simulink model "final_4_simu_20241216"  (R2021a)
settings: Solver=VariableStepAuto  StartTime=0.0  StopTime=30  RelTol=1e-3
model workspace (MAT data in the model file):
  x1_o = 0
values from neighbouring files (symbols this model uses):
  K = K_amp(1:3)    [plantilla_sscontrol.m]
  K_i = -K_amp(end)    [plantilla_sscontrol.m]
settings Model: Creator=juand  LastModifiedBy=frand

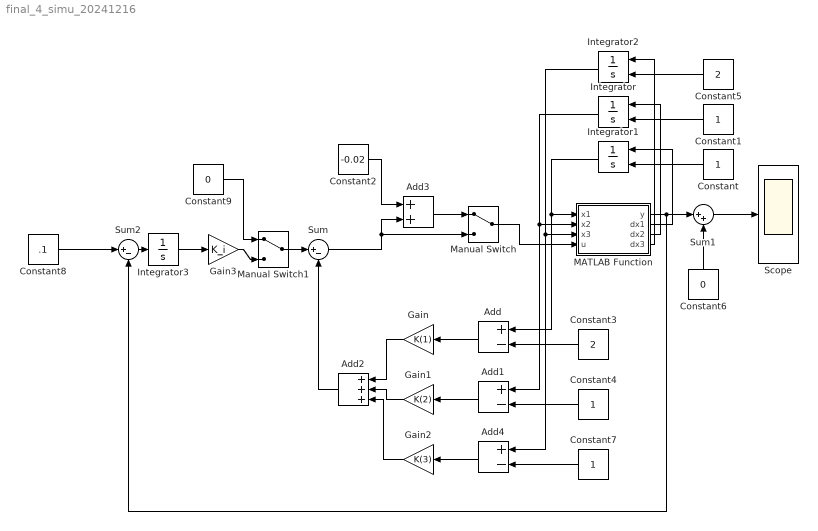
== system final_4_simu_20241216 ==
  Add : Sum  Inputs=+-
  Add1 : Sum  Inputs=+-
  Add2 : Sum  Inputs=+++
  Add3 : Sum
  Add4 : Sum  Inputs=+-
  Constant{,1,4,7} (4 alike) : Constant
  Constant2 : Constant  Value=-0.02
  Constant3 : Constant  Value=2
  Constant5 : Constant  Value=2
  Constant6 : Constant  Value=0
  Constant8 : Constant  Value=.1
  Constant9 : Constant  Value=0
  Gain : Gain  Gain=K(1)
  Gain1 : Gain  Gain=K(2)
  Gain2 : Gain  Gain=K(3)
  Gain3 : Gain  Gain=K_i
  Integrator : Integrator  InitialConditionSource=external  InitialCondition=x1_o
  Integrator1 : Integrator  InitialConditionSource=external
  Integrator2 : Integrator  InitialConditionSource=external  InitialCondition=x1_o
  Integrator3 : Integrator
  MATLAB Function : MATLAB Function  TreatAsAtomicUnit=on
  Manual Switch : ManualSwitch
  Manual Switch1 : ManualSwitch
  Scope : Scope
  Sum : Sum  Inputs=|+-
  Sum1 : Sum  Inputs=|++
  Sum2 : Sum  Inputs=|+-
  wires:
  MATLAB Function/2(dx1) -> Integrator1/1
  Integrator1/1 -> Add/1, MATLAB Function/1(x1)
  MATLAB Function/3(dx2) -> Integrator/1
  Integrator/1 -> Add1/1, MATLAB Function/2(x2)
  Constant/1 -> Integrator1/2
  Constant1/1 -> Integrator/2
  Add/1 -> Gain/1
  Add1/1 -> Gain1/1
  Constant3/1 -> Add/2
  Constant4/1 -> Add1/2
  Gain/1 -> Add2/1
  Gain1/1 -> Add2/2
  Add2/1 -> Sum/2
  Sum/1 -> Manual Switch/2, Add3/2
  Constant2/1 -> Add3/1
  Manual Switch/1 -> MATLAB Function/4(u)
  Add3/1 -> Manual Switch/1
  Integrator2/1 -> Add4/1, MATLAB Function/3(x3)
  MATLAB Function/4(dx3) -> Integrator2/1
  Constant5/1 -> Integrator2/2
  MATLAB Function/1(y) -> Sum1/1, Sum2/2
  Sum1/1 -> Scope/1
  Constant6/1 -> Sum1/2
  Constant7/1 -> Add4/2
  Add4/1 -> Gain2/1
  Gain2/1 -> Add2/3
  Constant8/1 -> Sum2/1
  Sum2/1 -> Integrator3/1
  Integrator3/1 -> Gain3/1
  Gain3/1 -> Manual Switch1/2
  Constant9/1 -> Manual Switch1/1
  Manual Switch1/1 -> Sum/1

== matlab function final_4_simu_20241216/MATLAB Function ==
  data: x1 input; x2 input; x3 input; u input; y output; dx1 output; dx2 output; dx3 output
function [y,dx1,dx2,dx3] = fcn(x1,x2,x3,u)

p = 0.02;

dx1 = (x3-sqrt(abs(x1-x2)))/(x1^2);
dx2 = (sqrt(abs(x1-x2))-sqrt(x2))/(x2^2);
dx3 = -p*x3+p*u;
y = x2;
